simulink model "multi_model2015a"  (R2015a)
settings: Solver=ode3  SolverMode=SingleTasking  StartTime=0.0  StopTime=inf  FixedStep=0.01  RelTol=1e-3
values from neighbouring files (symbols this model uses):
  s = serial (serPort)    [UART_Connector.m]
undefined symbols (not defined in the file or in its folder): deg, rad
libraries: simulink x12, aerolibconvert2 x2, aerolibobsolete x1, aerolibatmos2 x1, aerolibnav x1, aerolibanimutils x1
settings Model: Creator=ADAM  LastModifiedBy=theth
settings DataIOCC: MaxDataPoints=1  SaveFormat=Structure  SignalLoggingSaveFormat=ModelDataLogs  SaveOutput=off  SignalLogging=off  DSMLogging=off  SaveTime=off  OutputSaveName=model_out  SignalLoggingName=model_out
settings OptimizationCC: ExpressionDepthLimit=2147483647
settings DebuggingCC: UnderspecifiedInitializationDetection=Classic  MergeDetectMultiDrivingBlocksExec=none  SolverPrmCheckMsg=warning  MultiTaskDSMMsg=warning  MultiTaskCondExecSysMsg=none  StateNameClashWarn=warning
settings HardwareCC: ProdBitPerLong=64  ProdBitPerPointer=64  ProdIntDivRoundTo=Zero  ProdEndianess=LittleEndian  ProdWordSize=64  ProdHWDeviceType=Intel->x86-64  TargetBitPerLong=64  TargetBitPerPointer=64  TargetIntDivRoundTo=Zero  TargetEndianess=LittleEndian  TargetWordSize=64  TargetHWDeviceType=Intel->x86-64
settings ModelReferenceCC: EnableParallelModelReferenceBuilds=on
settings RTWCC: SystemTargetFile=rtwin.tlc  TemplateMakefile=rtwin.tmf  Description=Simulink Desktop Real-Time  RTWCompilerOptimization=on
settings CodeAppCC: MaxIdLength=95
settings RTWinTargetCC: TargetPreCompLibLocation=D:\Matlab\toolbox\sldrt\lib\win64  GeneratePreprocessorConditionals=Use local settings  UseToolchainInfoCompliant=off  ExtModeMexFile=sldrtext

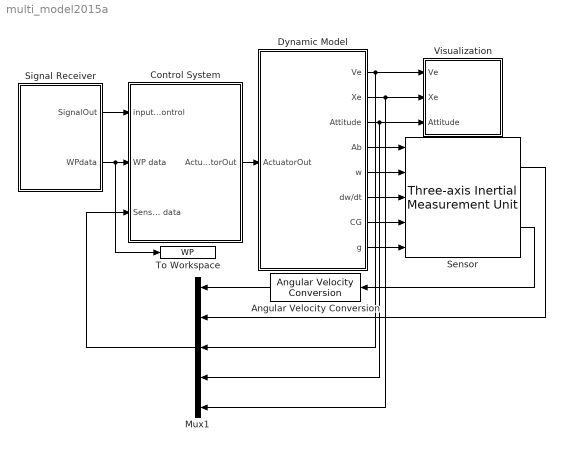
== system multi_model2015a ==
  Angular Velocity Conversion : aerolibconvert2/Angular Velocity Conversion  IU=rad/s  OU=deg/s
  Control System : Subsystem
      settings: CopyFcn=set_param(gcb,'BackgroundColor','green');
  Dynamic Model : Subsystem
      settings: CopyFcn=set_param(gcb,'BackgroundColor','orange');
  Mux1 : Mux  Inputs=5
  Sensor : aerolibnav/Three-axis Inertial Measurement Unit  units=Metric (MKS)  imu=[0 0 0]  dtype_a=off  w_a=190  z_a=0.707  a_sf_cc=[0.98 0 0; 0 0.98 0; 0 0 -0.98]  a_bias=[0 0 0]  a_sat="[-19.62  -19.62  -19.62 19.62 19.62 19.62]"  dtype_g=off  w_g=190  z_g=0.707  g_sf_cc=[.98 0 0; 0 .98 0; 0 0 .98]  g_bias=[0 0 0]  g_sens=[0 0 0]  g_sat="[-4.36  -4.36  -4.36 4.36 4.36 4.36]"  i_rand=on  i_seeds=[348631 366719 978432 189621 128794 214632]  i_pow=[0.000039 0.000039 0.000039 0.000000087 0.000000087 0.000000087]  i_Ts=0.01
  Signal Receiver : Subsystem
  To Workspace : ToWorkspace  VariableName=WP  SaveFormat=Structure  SampleTime=-1
  Visualization : Subsystem
  wires:
  Sensor/2 -> Angular Velocity Conversion/1
  Dynamic Model/2(Xe) -> Mux1/5, Visualization/2(Xe)
  Dynamic Model/3(Attitude) -> Mux1/4, Visualization/3(Attitude)
  Dynamic Model/4(Ab) -> Sensor/1
  Dynamic Model/5(w) -> Sensor/2
  Dynamic Model/6(dw/dt) -> Sensor/3
  Control System/1(ActuatorOut) -> Dynamic Model/1(ActuatorOut)
  Signal Receiver/1(SignalOut) -> Control System/1(inputControl)
  Dynamic Model/7(CG) -> Sensor/4
  Dynamic Model/8(g) -> Sensor/5
  Dynamic Model/1(Ve) -> Mux1/3, Visualization/1(Ve)
  Mux1/1 -> Control System/3(Sensors raw data)
  Angular Velocity Conversion/1 -> Mux1/1
  Sensor/1 -> Mux1/2
  Signal Receiver/2(WPdata) -> To Workspace/1, Control System/2(WP data)

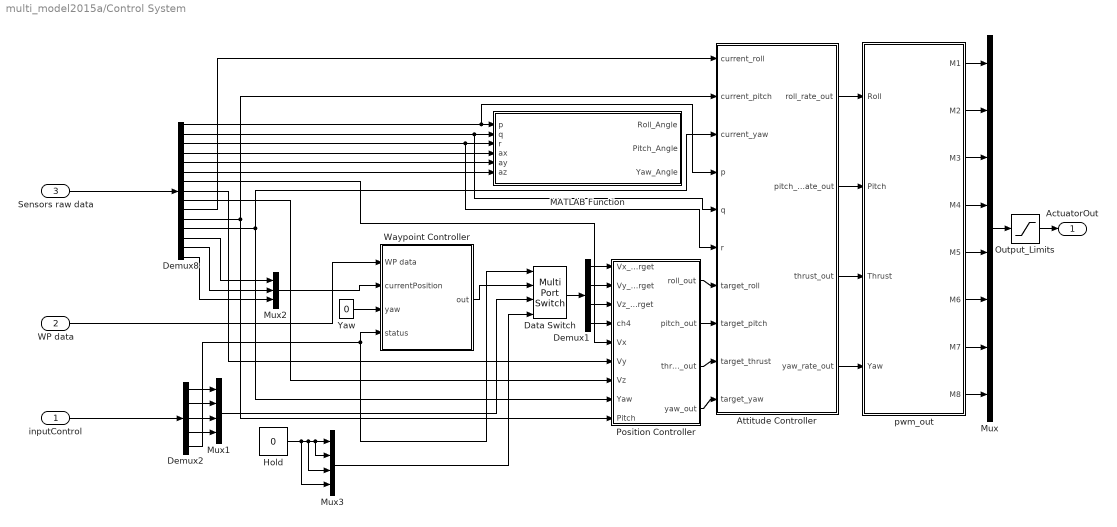
== system multi_model2015a/Control System ==
  inputControl : Inport
  WP data : Inport  Port=2
  Sensors raw data : Inport  Port=3
  Attitude Controller : Subsystem
  Data Switch : MultiPortSwitch  DataPortOrder=Zero-based contiguous
  Demux1 : Demux
  Demux2 : Demux  Outputs=5
  Demux8 : Demux  Outputs=15
  Hold : Constant  Value=0
  MATLAB Function : MATLAB Function  TreatAsAtomicUnit=on
      settings: PermitHierarchicalResolution=ParametersOnly
  Mux : Mux  Inputs=8
  Mux1 : Mux
  Mux2 : Mux  Inputs=3
  Mux3 : Mux
  Output_Limits : Saturate  UpperLimit=2000  LowerLimit=1000
  Position Controller : Subsystem
  Waypoint Controller : Subsystem
  Yaw : Constant  Value=0
  pwm_out : MATLAB Function  TreatAsAtomicUnit=on
      settings: PermitHierarchicalResolution=ParametersOnly
  ActuatorOut : Outport
  wires:
  pwm_out/8(M8) -> Mux/8
  pwm_out/7(M7) -> Mux/7
  pwm_out/6(M6) -> Mux/6
  pwm_out/5(M5) -> Mux/5
  pwm_out/4(M4) -> Mux/4
  pwm_out/3(M3) -> Mux/3
  pwm_out/2(M2) -> Mux/2
  pwm_out/1(M1) -> Mux/1
  Mux/1 -> Output_Limits/1
  Output_Limits/1 -> ActuatorOut/1
  Attitude Controller/3(thrust_out) -> pwm_out/3(Thrust)
  Attitude Controller/1(roll_rate_out) -> pwm_out/1(Roll)
  Attitude Controller/2(pitch_rate_out) -> pwm_out/2(Pitch)
  Attitude Controller/4(yaw_rate_out) -> pwm_out/4(Yaw)
  Position Controller/1(roll_out) -> Attitude Controller/7(target_roll)
  Position Controller/2(pitch_out) -> Attitude Controller/8(target_pitch)
  Position Controller/3(thrust_out) -> Attitude Controller/9(target_thrust)
  Position Controller/4(yaw_out) -> Attitude Controller/10(target_yaw)
  Demux1/3 -> Position Controller/3(Vz_target)
  Demux1/4 -> Position Controller/4(ch4)
  Demux1/1 -> Position Controller/1(Vx_target)
  Demux1/2 -> Position Controller/2(Vy_target)
  Demux8/1 -> Attitude Controller/4(p), MATLAB Function/1(p)
  Demux8/2 -> MATLAB Function/2(q), Attitude Controller/5(q)
  Demux8/3 -> MATLAB Function/3(r), Attitude Controller/6(r)
  Demux8/4 -> MATLAB Function/4(ax)
  Demux8/5 -> MATLAB Function/5(ay)
  Demux8/6 -> MATLAB Function/6(az)
  Demux8/7 -> Position Controller/5(Vx)
  Demux8/8 -> Position Controller/6(Vy)
  Demux8/9 -> Position Controller/7("Vz ")
  Demux8/12 -> Position Controller/8(Yaw), Attitude Controller/3(current_yaw)
  Demux8/11 -> Position Controller/9(Pitch), Attitude Controller/2(current_pitch)
  Demux8/10 -> Attitude Controller/1(current_roll)
  Yaw/1 -> Waypoint Controller/3(yaw)
  WP data/1 -> Waypoint Controller/1(WP data)
  Sensors raw data/1 -> Demux8/1
  Demux8/13 -> Mux2/1
  Demux8/14 -> Mux2/2
  Demux8/15 -> Mux2/3
  Mux2/1 -> Waypoint Controller/2(currentPosition)
  inputControl/1 -> Demux2/1
  Demux2/3 -> Mux1/3
  Demux2/2 -> Mux1/2
  Demux2/1 -> Mux1/1
  Demux2/4 -> Mux1/4
  Demux2/5 -> Data Switch/1, Waypoint Controller/4(status)
  Data Switch/1 -> Demux1/1
  Hold/1 -> Mux3/4, Mux3/3, Mux3/2, Mux3/1
  Mux3/1 -> Data Switch/4
  Waypoint Controller/1(out) -> Data Switch/2
  Mux1/1 -> Data Switch/3

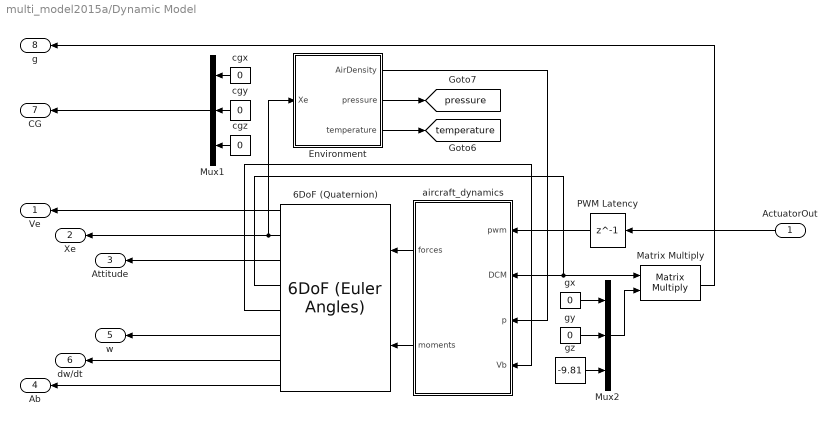
== system multi_model2015a/Dynamic Model ==
  ActuatorOut : Inport
  6DoF (Quaternion) : aerolibobsolete/6DoF (Euler Angles)  units=Metric (MKS)  mtype=Fixed  rep=Quaternion  xme_0=[0 0 0]  Vm_0=[0 0 0]  eul_0=[0 0 0]  pm_0=[0 0 0]  mass_0=1  mass_e=0  mass_f=0  inertia=[0.016, 0, 0; 0, 0.016, 0; 0, 0, 0.031]  inertia_e=eye(3)  inertia_f=eye(3)  k_quat=1.0
  Environment : Subsystem  TreatAsAtomicUnit=on
  Matrix Multiply : Product  Multiplication=Matrix(*)
  Mux1 : Mux  Inputs=3
  Mux2 : Mux  Inputs=3
  PWM Latency : Delay  DelayLength=1
  aircraft_dynamics : MATLAB Function  TreatAsAtomicUnit=on
      settings: PermitHierarchicalResolution=ParametersOnly
  cgx : Constant  Value=0
  cgy : Constant  Value=0
  cgz : Constant  Value=0
  gx : Constant  Value=0
  gy : Constant  Value=0
  gz : Constant  Value=-9.81
  Ve : Outport
  Xe : Outport  Port=2
  Attitude : Outport  Port=3
  Ab : Outport  Port=4
  w : Outport  Port=5
  dw/dt : Outport  Port=6
  CG : Outport  Port=7
  g : Outport  Port=8
  tag scope: pressure=global, temperature=global
  wires:
  6DoF (Quaternion)/4 -> Matrix Multiply/1, aircraft_dynamics/2(DCM)
  PWM Latency/1 -> aircraft_dynamics/1(pwm)
  6DoF (Quaternion)/2 -> Xe/1, Environment/1(Xe)
  6DoF (Quaternion)/5 -> aircraft_dynamics/4(Vb)
  aircraft_dynamics/2(moments) -> 6DoF (Quaternion)/2
  aircraft_dynamics/1(forces) -> 6DoF (Quaternion)/1
  6DoF (Quaternion)/6 -> w/1
  6DoF (Quaternion)/1 -> Ve/1
  6DoF (Quaternion)/3 -> Attitude/1
  Environment/1(AirDensity) -> aircraft_dynamics/3(p)
  Environment/3(temperature) -> [temperature]
  Environment/2(pressure) -> [pressure]
  ActuatorOut/1 -> PWM Latency/1
  6DoF (Quaternion)/8 -> Ab/1
  6DoF (Quaternion)/7 -> dw/dt/1
  cgy/1 -> Mux1/2
  gy/1 -> Mux2/2
  gx/1 -> Mux2/1
  cgx/1 -> Mux1/1
  cgz/1 -> Mux1/3
  gz/1 -> Mux2/3
  Mux2/1 -> Matrix Multiply/2
  Mux1/1 -> CG/1
  Matrix Multiply/1 -> g/1

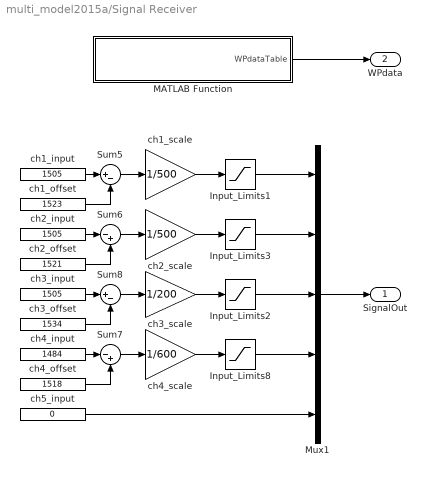
== system multi_model2015a/Signal Receiver ==
  Input_Limits1 : Saturate  UpperLimit=1  LowerLimit=-1
  Input_Limits2 : Saturate  UpperLimit=2.5  LowerLimit=-2.5
  Input_Limits3 : Saturate  UpperLimit=1  LowerLimit=-1
  Input_Limits8 : Saturate  UpperLimit=1  LowerLimit=-1
  MATLAB Function : MATLAB Function  TreatAsAtomicUnit=on
      settings: PermitHierarchicalResolution=ParametersOnly
  Mux1 : Mux  Inputs=5
  Sum5 : Sum  Inputs=|+-
  Sum6 : Sum  Inputs=|-+
  Sum7 : Sum  Inputs=|-+
  Sum8 : Sum  Inputs=|+-
  ch1_input : Constant  Value=1505
  ch1_offset : Constant  Value=1523
  ch1_scale : Gain  Gain=1/500
  ch2_input : Constant  Value=1505
  ch2_offset : Constant  Value=1521
  ch2_scale : Gain  Gain=1/500
  ch3_input : Constant  Value=1505
  ch3_offset : Constant  Value=1534
  ch3_scale : Gain  Gain=1/200
  ch4_input : Constant  Value=1484
  ch4_offset : Constant  Value=1518
  ch4_scale : Gain  Gain=1/600
  ch5_input : Constant  Value=0
  SignalOut : Outport
  WPdata : Outport  Port=2
  wires:
  Input_Limits8/1 -> Mux1/4
  Input_Limits2/1 -> Mux1/3
  Input_Limits1/1 -> Mux1/1
  Input_Limits3/1 -> Mux1/2
  Mux1/1 -> SignalOut/1
  MATLAB Function/1(WPdataTable) -> WPdata/1
  Sum6/1 -> ch2_scale/1
  Sum7/1 -> ch4_scale/1
  ch3_input/1 -> Sum8/1
  ch4_input/1 -> Sum7/1
  ch2_input/1 -> Sum6/1
  ch1_input/1 -> Sum5/1
  Sum5/1 -> ch1_scale/1
  Sum8/1 -> ch3_scale/1
  ch1_offset/1 -> Sum5/2
  ch2_offset/1 -> Sum6/2
  ch4_offset/1 -> Sum7/2
  ch4_scale/1 -> Input_Limits8/1
  ch3_offset/1 -> Sum8/2
  ch3_scale/1 -> Input_Limits2/1
  ch1_scale/1 -> Input_Limits1/1
  ch2_scale/1 -> Input_Limits3/1
  ch5_input/1 -> Mux1/5

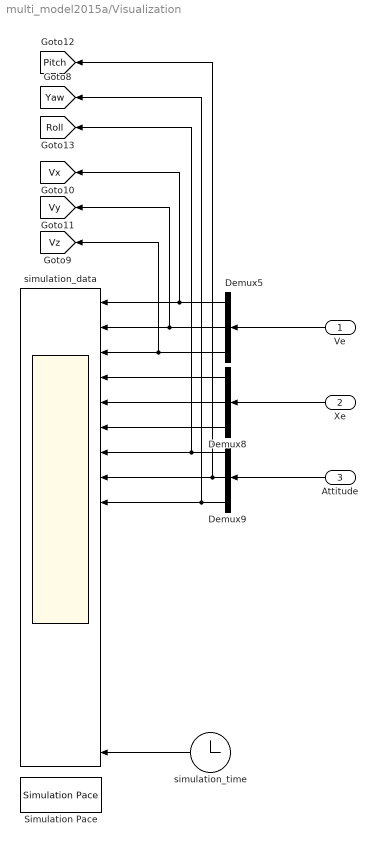
== system multi_model2015a/Visualization ==
  Ve : Inport
  Xe : Inport  Port=2
  Attitude : Inport  Port=3
  Demux5 : Demux  Outputs=3
  Demux8 : Demux  Outputs=3
  Demux9 : Demux  Outputs=3
  Simulation Pace : aerolibanimutils/Simulation Pace  SimulationPace=1  SleepMode=MATLAB Thread  OutputPaceError=off  SampleTime=-1
      settings: AttributesFormatString=%<SimulationPace> sec/sec
  simulation_data : Scope  NumInputPorts=19
      settings: TimeRange=auto  MaxDataPoints=5000  SaveToWorkspace=off  SaveName=ScopeData7  YMin=0.261~-0.28~15.25~34~-22~1725~-0.02~-0.04~0.01~-0.15~-0.1~-0.03~-0.4~-0.4~-10~-1~-5~-5~-5  YMax=0.275~-0.24~15.5~39~-17~1975~0.04~0.04~0.09~0.15~0.125~0.03~0.4~0.4~-9.2~1~5~5~5  SampleTime=-1
  simulation_time : Clock
  tag scope: Pitch=global, Roll=global, Vx=global, Vy=global, Vz=global, Yaw=global
  wires:
  Xe/1 -> Demux8/1
  Demux9/1 -> simulation_data/7, [Roll]
  Demux9/2 -> simulation_data/8, [Pitch]
  Attitude/1 -> Demux9/1
  Demux8/1 -> simulation_data/4
  Demux8/2 -> simulation_data/5
  Demux8/3 -> simulation_data/6
  Demux9/3 -> simulation_data/9, [Yaw]
  simulation_time/1 -> simulation_data/19
  Ve/1 -> Demux5/1
  Demux5/1 -> simulation_data/1, [Vx]
  Demux5/2 -> simulation_data/2, [Vy]
  Demux5/3 -> [Vz], simulation_data/3

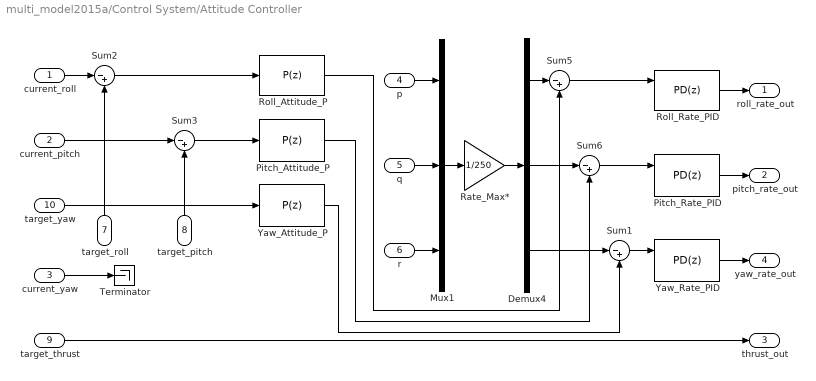
== system multi_model2015a/Control System/Attitude Controller ==
  current_roll : Inport
  current_pitch : Inport  Port=2
  current_yaw : Inport  Port=3
  p : Inport  Port=4
  q : Inport  Port=5
  r : Inport  Port=6
  target_roll : Inport  Port=7
  target_pitch : Inport  Port=8
  target_thrust : Inport  Port=9
  target_yaw : Inport  Port=10
  Demux4 : Demux  Outputs=3
  Mux1 : Mux  Inputs=3
  Pitch_Attitude_P : simulink/Continuous/PID Controller  Controller=P  TimeDomain=Discrete-time  SampleTime=-1  IntegratorMethod=Forward Euler  FilterMethod=Forward Euler  Form=Parallel  UseFilter=on  ControllerParametersSource=internal  P=1  I=0  D=0  N=100  InitialConditionSource=internal  InitialConditionForIntegrator=0  InitialConditionForFilter=0  ExternalReset=either  LimitOutput=on  UpperSaturationLimit=1  LowerSaturationLimit=-1  LinearizeAsGain=on  AntiWindupMode=none  Kb=1  TrackingMode=off  Kt=1  PParamMin=[]  PParamMax=[]  IParamMin=[]  IParamMax=[]  DParamMin=[]  DParamMax=[]  NParamMin=[]  NParamMax=[]  KbParamMin=[]  KbParamMax=[]  KtParamMin=[]  KtParamMax=[]  POutMin=[]  POutMax=[]  IOutMin=[]  IOutMax=[]  DOutMin=[]  DOutMax=[]  NOutMin=[]  NOutMax=[]  KbOutMin=[]  KbOutMax=[]  KtOutMin=[]  KtOutMax=[]  IntegratorOutMin=[]  IntegratorOutMax=[]  FilterOutMin=[]  FilterOutMax=[]  SumOutMin=[]  SumOutMax=[]  SumI1OutMin=[]  SumI1OutMax=[]  SumI2OutMin=[]  SumI2OutMax=[]  SumI3OutMin=[]  SumI3OutMax=[]  SumDOutMin=[]  SumDOutMax=[]  SaturationOutMin=[]  SaturationOutMax=[]  IntegratorContinuousStateAttributes=''  IntegratorStateMustResolveToSignalObject=off  IntegratorRTWStateStorageClass=Auto  FilterContinuousStateAttributes=''  FilterStateMustResolveToSignalObject=off  FilterRTWStateStorageClass=Auto  DifferentiatorICPrevScaledInput=0  DifferentiatorOutMin=[]  DifferentiatorOutMax=[]
  Pitch_Rate_PID : simulink/Continuous/PID Controller  Controller=PD  TimeDomain=Discrete-time  SampleTime=-1  IntegratorMethod=Forward Euler  FilterMethod=Forward Euler  Form=Parallel  UseFilter=off  ControllerParametersSource=internal  P=2  I=0  D=0.01  N=20  InitialConditionSource=internal  InitialConditionForIntegrator=0  InitialConditionForFilter=0  ExternalReset=either  LimitOutput=on  UpperSaturationLimit=1  LowerSaturationLimit=-1  LinearizeAsGain=on  AntiWindupMode=none  Kb=1  TrackingMode=off  Kt=1  PParamMin=[]  PParamMax=[]  IParamMin=[]  IParamMax=[]  DParamMin=[]  DParamMax=[]  NParamMin=[]  NParamMax=[]  KbParamMin=[]  KbParamMax=[]  KtParamMin=[]  KtParamMax=[]  POutMin=[]  POutMax=[]  IOutMin=[]  IOutMax=[]  DOutMin=[]  DOutMax=[]  NOutMin=[]  NOutMax=[]  KbOutMin=[]  KbOutMax=[]  KtOutMin=[]  KtOutMax=[]  IntegratorOutMin=[]  IntegratorOutMax=[]  FilterOutMin=[]  FilterOutMax=[]  SumOutMin=[]  SumOutMax=[]  SumI1OutMin=[]  SumI1OutMax=[]  SumI2OutMin=[]  SumI2OutMax=[]  SumI3OutMin=[]  SumI3OutMax=[]  SumDOutMin=[]  SumDOutMax=[]  SaturationOutMin=[]  SaturationOutMax=[]  IntegratorContinuousStateAttributes=''  IntegratorStateMustResolveToSignalObject=off  IntegratorRTWStateStorageClass=Auto  FilterContinuousStateAttributes=''  FilterStateMustResolveToSignalObject=off  FilterRTWStateStorageClass=Auto  DifferentiatorICPrevScaledInput=0  DifferentiatorOutMin=[]  DifferentiatorOutMax=[]
  Rate_Max* : Gain  Gain=1/250
  Roll_Attitude_P : simulink/Continuous/PID Controller  Controller=P  TimeDomain=Discrete-time  SampleTime=-1  IntegratorMethod=Forward Euler  FilterMethod=Forward Euler  Form=Parallel  UseFilter=on  ControllerParametersSource=internal  P=1  I=0  D=0  N=100  InitialConditionSource=internal  InitialConditionForIntegrator=0  InitialConditionForFilter=0  ExternalReset=either  LimitOutput=on  UpperSaturationLimit=1  LowerSaturationLimit=-1  LinearizeAsGain=on  AntiWindupMode=none  Kb=1  TrackingMode=off  Kt=1  PParamMin=[]  PParamMax=[]  IParamMin=[]  IParamMax=[]  DParamMin=[]  DParamMax=[]  NParamMin=[]  NParamMax=[]  KbParamMin=[]  KbParamMax=[]  KtParamMin=[]  KtParamMax=[]  POutMin=[]  POutMax=[]  IOutMin=[]  IOutMax=[]  DOutMin=[]  DOutMax=[]  NOutMin=[]  NOutMax=[]  KbOutMin=[]  KbOutMax=[]  KtOutMin=[]  KtOutMax=[]  IntegratorOutMin=[]  IntegratorOutMax=[]  FilterOutMin=[]  FilterOutMax=[]  SumOutMin=[]  SumOutMax=[]  SumI1OutMin=[]  SumI1OutMax=[]  SumI2OutMin=[]  SumI2OutMax=[]  SumI3OutMin=[]  SumI3OutMax=[]  SumDOutMin=[]  SumDOutMax=[]  SaturationOutMin=[]  SaturationOutMax=[]  IntegratorContinuousStateAttributes=''  IntegratorStateMustResolveToSignalObject=off  IntegratorRTWStateStorageClass=Auto  FilterContinuousStateAttributes=''  FilterStateMustResolveToSignalObject=off  FilterRTWStateStorageClass=Auto  DifferentiatorICPrevScaledInput=0  DifferentiatorOutMin=[]  DifferentiatorOutMax=[]
  Roll_Rate_PID : simulink/Continuous/PID Controller  Controller=PD  TimeDomain=Discrete-time  SampleTime=-1  IntegratorMethod=Forward Euler  FilterMethod=Forward Euler  Form=Parallel  UseFilter=off  ControllerParametersSource=internal  P=2  I=0  D=0.01  N=20  InitialConditionSource=internal  InitialConditionForIntegrator=0  InitialConditionForFilter=0  ExternalReset=either  LimitOutput=on  UpperSaturationLimit=1  LowerSaturationLimit=-1  LinearizeAsGain=on  AntiWindupMode=none  Kb=1  TrackingMode=off  Kt=1  PParamMin=[]  PParamMax=[]  IParamMin=[]  IParamMax=[]  DParamMin=[]  DParamMax=[]  NParamMin=[]  NParamMax=[]  KbParamMin=[]  KbParamMax=[]  KtParamMin=[]  KtParamMax=[]  POutMin=[]  POutMax=[]  IOutMin=[]  IOutMax=[]  DOutMin=[]  DOutMax=[]  NOutMin=[]  NOutMax=[]  KbOutMin=[]  KbOutMax=[]  KtOutMin=[]  KtOutMax=[]  IntegratorOutMin=[]  IntegratorOutMax=[]  FilterOutMin=[]  FilterOutMax=[]  SumOutMin=[]  SumOutMax=[]  SumI1OutMin=[]  SumI1OutMax=[]  SumI2OutMin=[]  SumI2OutMax=[]  SumI3OutMin=[]  SumI3OutMax=[]  SumDOutMin=[]  SumDOutMax=[]  SaturationOutMin=[]  SaturationOutMax=[]  IntegratorContinuousStateAttributes=''  IntegratorStateMustResolveToSignalObject=off  IntegratorRTWStateStorageClass=Auto  FilterContinuousStateAttributes=''  FilterStateMustResolveToSignalObject=off  FilterRTWStateStorageClass=Auto  DifferentiatorICPrevScaledInput=0  DifferentiatorOutMin=[]  DifferentiatorOutMax=[]
  Sum{1..3,5..6} (5 alike) : Sum  Inputs=|-+
  Terminator : Terminator
  Yaw_Attitude_P : simulink/Continuous/PID Controller  Controller=P  TimeDomain=Discrete-time  SampleTime=-1  IntegratorMethod=Forward Euler  FilterMethod=Forward Euler  Form=Parallel  UseFilter=on  ControllerParametersSource=internal  P=1  I=0  D=0  N=100  InitialConditionSource=internal  InitialConditionForIntegrator=0  InitialConditionForFilter=0  ExternalReset=either  LimitOutput=on  UpperSaturationLimit=1  LowerSaturationLimit=-1  LinearizeAsGain=on  AntiWindupMode=none  Kb=1  TrackingMode=off  Kt=1  PParamMin=[]  PParamMax=[]  IParamMin=[]  IParamMax=[]  DParamMin=[]  DParamMax=[]  NParamMin=[]  NParamMax=[]  KbParamMin=[]  KbParamMax=[]  KtParamMin=[]  KtParamMax=[]  POutMin=[]  POutMax=[]  IOutMin=[]  IOutMax=[]  DOutMin=[]  DOutMax=[]  NOutMin=[]  NOutMax=[]  KbOutMin=[]  KbOutMax=[]  KtOutMin=[]  KtOutMax=[]  IntegratorOutMin=[]  IntegratorOutMax=[]  FilterOutMin=[]  FilterOutMax=[]  SumOutMin=[]  SumOutMax=[]  SumI1OutMin=[]  SumI1OutMax=[]  SumI2OutMin=[]  SumI2OutMax=[]  SumI3OutMin=[]  SumI3OutMax=[]  SumDOutMin=[]  SumDOutMax=[]  SaturationOutMin=[]  SaturationOutMax=[]  IntegratorContinuousStateAttributes=''  IntegratorStateMustResolveToSignalObject=off  IntegratorRTWStateStorageClass=Auto  FilterContinuousStateAttributes=''  FilterStateMustResolveToSignalObject=off  FilterRTWStateStorageClass=Auto  DifferentiatorICPrevScaledInput=0  DifferentiatorOutMin=[]  DifferentiatorOutMax=[]
  Yaw_Rate_PID : simulink/Continuous/PID Controller  Controller=PD  TimeDomain=Discrete-time  SampleTime=-1  IntegratorMethod=Forward Euler  FilterMethod=Forward Euler  Form=Parallel  UseFilter=off  ControllerParametersSource=internal  P=4.5  I=0  D=0.1  N=20  InitialConditionSource=internal  InitialConditionForIntegrator=0  InitialConditionForFilter=0  ExternalReset=either  LimitOutput=on  UpperSaturationLimit=1  LowerSaturationLimit=-1  LinearizeAsGain=on  AntiWindupMode=none  Kb=1  TrackingMode=off  Kt=1  PParamMin=[]  PParamMax=[]  IParamMin=[]  IParamMax=[]  DParamMin=[]  DParamMax=[]  NParamMin=[]  NParamMax=[]  KbParamMin=[]  KbParamMax=[]  KtParamMin=[]  KtParamMax=[]  POutMin=[]  POutMax=[]  IOutMin=[]  IOutMax=[]  DOutMin=[]  DOutMax=[]  NOutMin=[]  NOutMax=[]  KbOutMin=[]  KbOutMax=[]  KtOutMin=[]  KtOutMax=[]  IntegratorOutMin=[]  IntegratorOutMax=[]  FilterOutMin=[]  FilterOutMax=[]  SumOutMin=[]  SumOutMax=[]  SumI1OutMin=[]  SumI1OutMax=[]  SumI2OutMin=[]  SumI2OutMax=[]  SumI3OutMin=[]  SumI3OutMax=[]  SumDOutMin=[]  SumDOutMax=[]  SaturationOutMin=[]  SaturationOutMax=[]  IntegratorContinuousStateAttributes=''  IntegratorStateMustResolveToSignalObject=off  IntegratorRTWStateStorageClass=Auto  FilterContinuousStateAttributes=''  FilterStateMustResolveToSignalObject=off  FilterRTWStateStorageClass=Auto  DifferentiatorICPrevScaledInput=0  DifferentiatorOutMin=[]  DifferentiatorOutMax=[]
  roll_rate_out : Outport
  pitch_rate_out : Outport  Port=2
  thrust_out : Outport  Port=3
  yaw_rate_out : Outport  Port=4
  wires:
  Sum5/1 -> Roll_Rate_PID/1
  Rate_Max*/1 -> Demux4/1
  Demux4/2 -> Sum6/1
  Demux4/1 -> Sum5/1
  Sum1/1 -> Yaw_Rate_PID/1
  Sum6/1 -> Pitch_Rate_PID/1
  Demux4/3 -> Sum1/1
  Mux1/1 -> Rate_Max*/1
  Sum2/1 -> Roll_Attitude_P/1
  Sum3/1 -> Pitch_Attitude_P/1
  current_pitch/1 -> Sum3/1
  current_roll/1 -> Sum2/1
  p/1 -> Mux1/1
  q/1 -> Mux1/2
  r/1 -> Mux1/3
  Yaw_Attitude_P/1 -> Sum1/2
  Pitch_Attitude_P/1 -> Sum6/2
  Roll_Attitude_P/1 -> Sum5/2
  target_roll/1 -> Sum2/2
  target_pitch/1 -> Sum3/2
  target_thrust/1 -> thrust_out/1
  Yaw_Rate_PID/1 -> yaw_rate_out/1
  Pitch_Rate_PID/1 -> pitch_rate_out/1
  Roll_Rate_PID/1 -> roll_rate_out/1
  target_yaw/1 -> Yaw_Attitude_P/1
  current_yaw/1 -> Terminator/1

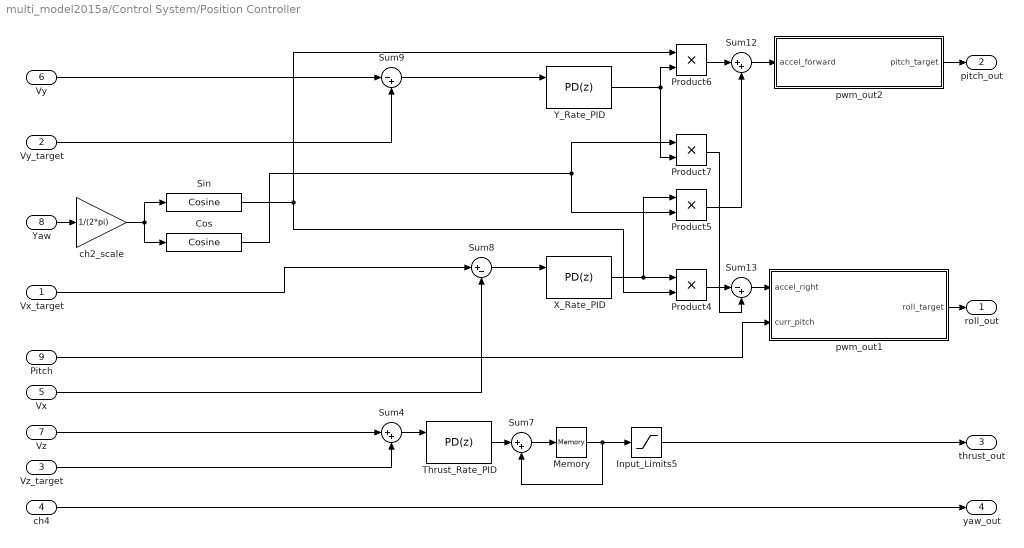
== system multi_model2015a/Control System/Position Controller ==
  Vx_target : Inport
  Vy_target : Inport  Port=2
  Vz_target : Inport  Port=3
  ch4 : Inport  Port=4
  Vx : Inport  Port=5
  Vy : Inport  Port=6
  "Vz " : Inport  Port=7
  Yaw : Inport  Port=8
  Pitch : Inport  Port=9
  Cos : simulink/Lookup Tables/Cosine  Formula=cos(2*pi*u)  NumDataPoints=(2^5)+1  OutputWordLength=16  InternalRulePriority=Speed
  Input_Limits5 : Saturate  UpperLimit=1  LowerLimit=0
  Memory : Memory  InheritSampleTime=on  LinearizeMemory=on
  Product{4..7} (4 alike) : Product
  Sin : simulink/Lookup Tables/Cosine  Formula=sin(2*pi*u)  NumDataPoints=(2^5)+1  OutputWordLength=16  InternalRulePriority=Speed
  Sum12 : Sum  Inputs=|++
  Sum13 : Sum  Inputs=|-+
  Sum4 : Sum  Inputs=|++
  Sum7 : Sum  Inputs=|++
  Sum8 : Sum  Inputs=|+-
  Sum9 : Sum  Inputs=|-+
  Thrust_Rate_PID : simulink/Continuous/PID Controller  Controller=PD  TimeDomain=Discrete-time  SampleTime=-1  IntegratorMethod=Forward Euler  FilterMethod=Forward Euler  Form=Parallel  UseFilter=off  ControllerParametersSource=internal  P=0.1  I=0.1  D=0.01  N=20  InitialConditionSource=internal  InitialConditionForIntegrator=0  InitialConditionForFilter=0  ExternalReset=either  LimitOutput=on  UpperSaturationLimit=1  LowerSaturationLimit=-1  LinearizeAsGain=on  AntiWindupMode=none  Kb=1  TrackingMode=off  Kt=1  PParamMin=[]  PParamMax=[]  IParamMin=[]  IParamMax=[]  DParamMin=[]  DParamMax=[]  NParamMin=[]  NParamMax=[]  KbParamMin=[]  KbParamMax=[]  KtParamMin=[]  KtParamMax=[]  POutMin=[]  POutMax=[]  IOutMin=[]  IOutMax=[]  DOutMin=[]  DOutMax=[]  NOutMin=[]  NOutMax=[]  KbOutMin=[]  KbOutMax=[]  KtOutMin=[]  KtOutMax=[]  IntegratorOutMin=[]  IntegratorOutMax=[]  FilterOutMin=[]  FilterOutMax=[]  SumOutMin=[]  SumOutMax=[]  SumI1OutMin=[]  SumI1OutMax=[]  SumI2OutMin=[]  SumI2OutMax=[]  SumI3OutMin=[]  SumI3OutMax=[]  SumDOutMin=[]  SumDOutMax=[]  SaturationOutMin=[]  SaturationOutMax=[]  IntegratorContinuousStateAttributes=''  IntegratorStateMustResolveToSignalObject=off  IntegratorRTWStateStorageClass=Auto  FilterContinuousStateAttributes=''  FilterStateMustResolveToSignalObject=off  FilterRTWStateStorageClass=Auto  DifferentiatorICPrevScaledInput=0  DifferentiatorOutMin=[]  DifferentiatorOutMax=[]
  X_Rate_PID : simulink/Continuous/PID Controller  Controller=PD  TimeDomain=Discrete-time  SampleTime=-1  IntegratorMethod=Forward Euler  FilterMethod=Forward Euler  Form=Parallel  UseFilter=off  ControllerParametersSource=internal  P=1  I=0.01  D=0.01  N=20  InitialConditionSource=internal  InitialConditionForIntegrator=0  InitialConditionForFilter=0  ExternalReset=either  LimitOutput=on  UpperSaturationLimit=1  LowerSaturationLimit=-1  LinearizeAsGain=on  AntiWindupMode=none  Kb=1  TrackingMode=off  Kt=1  PParamMin=[]  PParamMax=[]  IParamMin=[]  IParamMax=[]  DParamMin=[]  DParamMax=[]  NParamMin=[]  NParamMax=[]  KbParamMin=[]  KbParamMax=[]  KtParamMin=[]  KtParamMax=[]  POutMin=[]  POutMax=[]  IOutMin=[]  IOutMax=[]  DOutMin=[]  DOutMax=[]  NOutMin=[]  NOutMax=[]  KbOutMin=[]  KbOutMax=[]  KtOutMin=[]  KtOutMax=[]  IntegratorOutMin=[]  IntegratorOutMax=[]  FilterOutMin=[]  FilterOutMax=[]  SumOutMin=[]  SumOutMax=[]  SumI1OutMin=[]  SumI1OutMax=[]  SumI2OutMin=[]  SumI2OutMax=[]  SumI3OutMin=[]  SumI3OutMax=[]  SumDOutMin=[]  SumDOutMax=[]  SaturationOutMin=[]  SaturationOutMax=[]  IntegratorContinuousStateAttributes=''  IntegratorStateMustResolveToSignalObject=off  IntegratorRTWStateStorageClass=Auto  FilterContinuousStateAttributes=''  FilterStateMustResolveToSignalObject=off  FilterRTWStateStorageClass=Auto  DifferentiatorICPrevScaledInput=0  DifferentiatorOutMin=[]  DifferentiatorOutMax=[]
  Y_Rate_PID : simulink/Continuous/PID Controller  Controller=PD  TimeDomain=Discrete-time  SampleTime=-1  IntegratorMethod=Forward Euler  FilterMethod=Forward Euler  Form=Parallel  UseFilter=off  ControllerParametersSource=internal  P=1  I=0.01  D=0.01  N=20  InitialConditionSource=internal  InitialConditionForIntegrator=0  InitialConditionForFilter=0  ExternalReset=either  LimitOutput=on  UpperSaturationLimit=1  LowerSaturationLimit=-1  LinearizeAsGain=on  AntiWindupMode=none  Kb=1  TrackingMode=off  Kt=1  PParamMin=[]  PParamMax=[]  IParamMin=[]  IParamMax=[]  DParamMin=[]  DParamMax=[]  NParamMin=[]  NParamMax=[]  KbParamMin=[]  KbParamMax=[]  KtParamMin=[]  KtParamMax=[]  POutMin=[]  POutMax=[]  IOutMin=[]  IOutMax=[]  DOutMin=[]  DOutMax=[]  NOutMin=[]  NOutMax=[]  KbOutMin=[]  KbOutMax=[]  KtOutMin=[]  KtOutMax=[]  IntegratorOutMin=[]  IntegratorOutMax=[]  FilterOutMin=[]  FilterOutMax=[]  SumOutMin=[]  SumOutMax=[]  SumI1OutMin=[]  SumI1OutMax=[]  SumI2OutMin=[]  SumI2OutMax=[]  SumI3OutMin=[]  SumI3OutMax=[]  SumDOutMin=[]  SumDOutMax=[]  SaturationOutMin=[]  SaturationOutMax=[]  IntegratorContinuousStateAttributes=''  IntegratorStateMustResolveToSignalObject=off  IntegratorRTWStateStorageClass=Auto  FilterContinuousStateAttributes=''  FilterStateMustResolveToSignalObject=off  FilterRTWStateStorageClass=Auto  DifferentiatorICPrevScaledInput=0  DifferentiatorOutMin=[]  DifferentiatorOutMax=[]
  ch2_scale : Gain  Gain=1/(2*pi)
  pwm_out1 : MATLAB Function  TreatAsAtomicUnit=on
      settings: PermitHierarchicalResolution=ParametersOnly
  pwm_out2 : MATLAB Function  TreatAsAtomicUnit=on
      settings: PermitHierarchicalResolution=ParametersOnly
  roll_out : Outport
  pitch_out : Outport  Port=2
  thrust_out : Outport  Port=3
  yaw_out : Outport  Port=4
  wires:
  X_Rate_PID/1 -> Product4/1, Product5/1
  Y_Rate_PID/1 -> Product7/2, Product6/2
  Sum8/1 -> X_Rate_PID/1
  Vx_target/1 -> Sum8/1
  Sum12/1 -> pwm_out2/1(accel_forward)
  Cos/1 -> Product7/1, Product5/2
  Sin/1 -> Product6/1, Product4/2
  Yaw/1 -> ch2_scale/1
  Vy/1 -> Sum9/1
  Sum9/1 -> Y_Rate_PID/1
  Vx/1 -> Sum8/2
  pwm_out2/1(pitch_target) -> pitch_out/1
  pwm_out1/1(roll_target) -> roll_out/1
  ch4/1 -> yaw_out/1
  Product5/1 -> Sum12/2
  Product6/1 -> Sum12/1
  Sum13/1 -> pwm_out1/1(accel_right)
  Pitch/1 -> pwm_out1/2(curr_pitch)
  Product7/1 -> Sum13/2
  Product4/1 -> Sum13/1
  ch2_scale/1 -> Cos/1, Sin/1
  Sum4/1 -> Thrust_Rate_PID/1
  Memory/1 -> Input_Limits5/1, Sum7/2
  Sum7/1 -> Memory/1
  Thrust_Rate_PID/1 -> Sum7/1
  "Vz "/1 -> Sum4/1
  Vz_target/1 -> Sum4/2
  Input_Limits5/1 -> thrust_out/1
  Vy_target/1 -> Sum9/2

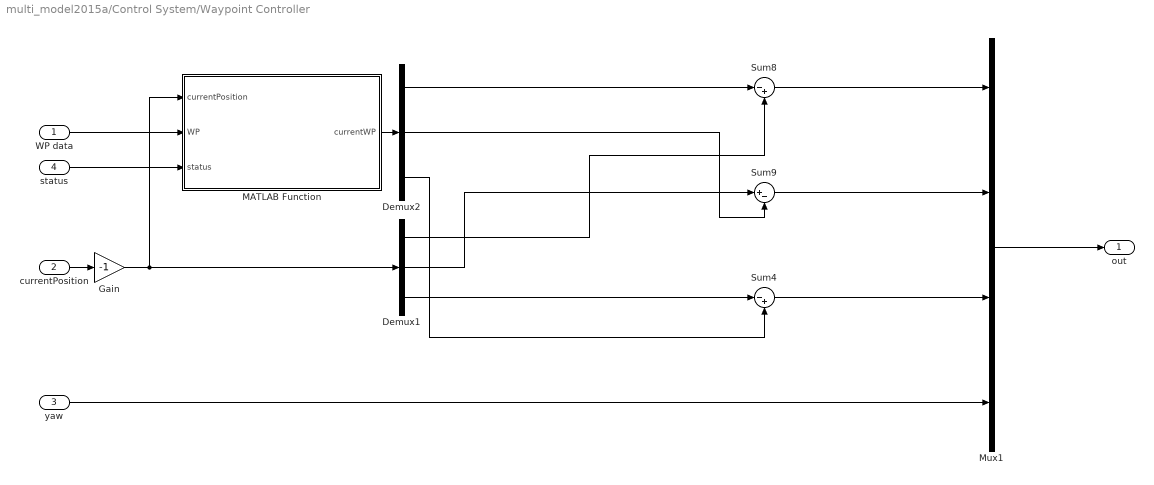
== system multi_model2015a/Control System/Waypoint Controller ==
  WP data : Inport
  currentPosition : Inport  Port=2
  yaw : Inport  Port=3
  status : Inport  Port=4
  Demux1 : Demux  Outputs=3
  Demux2 : Demux  Outputs=3
  Gain : Gain  Gain=-1
  MATLAB Function : MATLAB Function  TreatAsAtomicUnit=on
      settings: PermitHierarchicalResolution=ParametersOnly
  Mux1 : Mux
  Sum4 : Sum  Inputs=|-+
  Sum8 : Sum  Inputs=|-+
  Sum9 : Sum  Inputs=|+-
  out : Outport
  wires:
  Demux2/1 -> Sum8/1
  Demux1/2 -> Sum9/1
  Demux1/1 -> Sum8/2
  yaw/1 -> Mux1/4
  Demux1/3 -> Sum4/1
  Demux2/3 -> Sum4/2
  Mux1/1 -> out/1
  MATLAB Function/1(currentWP) -> Demux2/1
  Demux2/2 -> Sum9/2
  WP data/1 -> MATLAB Function/2(WP)
  status/1 -> MATLAB Function/3(status)
  Sum9/1 -> Mux1/2
  Sum4/1 -> Mux1/3
  Sum8/1 -> Mux1/1
  currentPosition/1 -> Gain/1
  Gain/1 -> MATLAB Function/1(currentPosition), Demux1/1

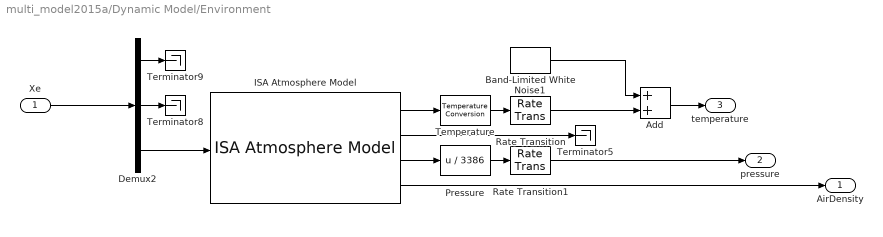
== system multi_model2015a/Dynamic Model/Environment ==
  Xe : Inport
  Add : Sum
  Band-Limited White Noise1 : simulink/Sources/Band-Limited White Noise  Cov=[0.0001]  Ts=0.5  seed=[23341]
  Demux2 : Demux  Outputs=3
  ISA Atmosphere Model : aerolibatmos2/ISA Atmosphere Model  custom=on  g=9.80665  gamma=1.4  R=287.0531  L=0.0065  h_trop=11000  h_strat=20000  rho0=1.225  P0=101325  T0=288.15  h0=0
  Pressure : Fcn  Expr=u / 3386
  Rate Transition : RateTransition  OutPortSampleTime=0.01
  Rate Transition1 : RateTransition  OutPortSampleTime=0.05
  Temperature : aerolibconvert2/Temperature Conversion  IU=K  OU=C
  Terminator5 : Terminator
  Terminator8 : Terminator
  Terminator9 : Terminator
  AirDensity : Outport
  pressure : Outport  Port=2
  temperature : Outport  Port=3
  wires:
  Demux2/2 -> Terminator8/1
  Demux2/1 -> Terminator9/1
  Demux2/3 -> ISA Atmosphere Model/1
  Xe/1 -> Demux2/1
  ISA Atmosphere Model/3 -> Pressure/1
  ISA Atmosphere Model/2 -> Terminator5/1
  ISA Atmosphere Model/4 -> AirDensity/1
  ISA Atmosphere Model/1 -> Temperature/1
  Temperature/1 -> Rate Transition/1
  Pressure/1 -> Rate Transition1/1
  Rate Transition/1 -> Add/2
  Add/1 -> temperature/1
  Rate Transition1/1 -> pressure/1
  Band-Limited White Noise1/1 -> Add/1

== matlab function multi_model2015a/Control System/MATLAB Function ==
  data: p input; q input; r input; ax input; ay input; az input; Roll_Angle output; Pitch_Angle output; Yaw_Angle output
function [Roll_Angle, Pitch_Angle, Yaw_Angle] = sensor_fusion(p, q, r, ax, ay, az)

%================================Constants=================================

delta_t = 0.01;
degrees = 180 / pi;
radians = pi / 180;

%Attitude Estimator
Q_gyroBias = 0.000000087;           % Q_gyroBias: gyroscope noise
Q_angle = 0.000039;                 % Q_angle: accelerometer noise
R_angle = 20;                       % R_angle: high ==> gyroscope, low ==> accelerometer

%=============================Intitialization==============================

persistent initialize angle_roll bias1 P1 K1 phi angle_pitch bias2 P2 K2 theta angle_yaw;
    
if isempty(initialize)
    if isempty(angle_roll)
        angle_roll = 0;
        bias1 = 0;
        P1 = zeros(2);
        K1 = zeros([2,1]);
        phi = 0;
    end
    if isempty(angle_pitch)
        angle_pitch = 0;
        bias2 = 0;
        P2 = zeros(2);
        K2 = zeros([2,1]);
        theta = 0;
    end
    if isempty(angle_yaw)
        angle_yaw = 0;
    end
    initialize = 1;
else
    
%==============================Kalman Filter===============================

%--------------------------------Roll Angle--------------------------------

    Rate_Roll = p + (q * sin(phi) + r * cos(phi)) * tan(theta) - bias1;                     
    angle_roll = angle_roll + Rate_Roll * delta_t;                                          %Projected State (integrated gyro data)
    earth_roll = -atan(ay / az) * degrees;                                                  %Measurement Update (gravity vector)
    P1(1,1) = P1(1,1) + delta_t * (P1(2,2) * delta_t - P1(1,2) - P1(2,1) + Q_angle);        %Projected error covariance
    P1(1,2) = P1(1,2) - P1(2,2) * delta_t;
    P1(2,1) = P1(2,1) - P1(2,2) * delta_t;
    P1(2,2) = P1(2,2) + Q_gyroBias * delta_t;
    S1 = P1(1,1) + R_angle;                                                                 %Kalman Gain
    K1(1) = P1(1,1) / S1;
    K1(2) = P1(2,1) / S1;
    Y1 = earth_roll - angle_roll;                                                           %Estimate Update
    angle_roll = angle_roll + K1(1) * Y1;
    bias1 = bias1 + K1(2) * Y1;
    P1(1,1) = P1(1,1) - K1(1) * P1(1,1);                                                    %Update Error Covariance
    P1(1,2) = P1(1,2) - K1(1) * P1(1,2);
    P1(2,1) = P1(2,1) - K1(2) * P1(1,1);
    P1(2,2) = P1(2,2) - K1(2) * P1(1,2);
    phi = angle_roll * radians;
 
%--------------------------------Pitch Angle-------------------------------

    Rate_Pitch = q * cos(phi) + r * sin(phi) - bias2;                           
    angle_pitch = angle_pitch + Rate_Pitch * delta_t;                                       %Projected State (integrated gyro data)
    earth_pitch = atan(ax / az) * degrees;                                                  %Measurement Update (gravity vector)
    P2(1,1) = P2(1,1) + delta_t * (P2(2,2) * delta_t - P2(1,2) - P2(2,1) + Q_angle);        %Projected error covariance
    P2(1,2) = P2(1,2) - P2(2,2) * delta_t;
    P2(2,1) = P2(2,1) - P2(2,2) * delta_t;
    P2(2,2) = P2(2,2) + Q_gyroBias * delta_t;
    S2 = P2(1,1) + R_angle;                                                                 %Kalman Gain
    K2(1) = P2(1,1) / S2;
    K2(2) = P2(2,1) / S2;
    Y2 = earth_pitch - angle_pitch;                                                         %Estimate Update
    angle_pitch = angle_pitch + K2(1) * Y2;
    bias2 = bias2 + K2(2) * Y2;
    P2(1,1) = P2(1,1) - K2(1) * P2(1,1);                                                    %Update Error Covariance
    P2(1,2) = P2(1,2) - K2(1) * P2(1,2);
    P2(2,1) = P2(2,1) - K2(2) * P2(1,1);
    P2(2,2) = P2(2,2) - K2(2) * P2(1,2);
    theta = angle_pitch * radians;
    
%--------------------------------Yaw Angle---------------------------------

    angle_yaw = angle_yaw + (q * sin(phi) + r * cos(phi)) * sec(theta) * delta_t;           %Integrated gyro data

end

Roll_Angle = phi;
Pitch_Angle = theta;
Yaw_Angle = angle_yaw * radians/(2*pi);
    
%==========================================================================

== matlab function multi_model2015a/Control System/Waypoint Controller/MATLAB Function ==
  data: currentPosition input; WP input; status input; currentWP output
function currentWP = currentWP(currentPosition, WP, status)
%=============================Intitialization==============================
persistent initialize index sizeWPArray;
    
if isempty(initialize)
    if isempty(index)
        index = 1;       
    end    
    sizeWPArray = length(WP(:,1));  
    initialize = 1;
else
    if(status == 0)
        if((norm(-transpose(currentPosition) + WP(index,:)) < 0.1) && (index < sizeWPArray))
        index = index + 1;
        end   
    end
end
currentWP = WP(index,:);

== matlab function multi_model2015a/Control System/Position Controller/pwm_out1 ==
  data: accel_right input; curr_pitch input; roll_target output
function roll_target  = accel2roll_target(accel_right, curr_pitch)
roll_target = atan(accel_right*cos(curr_pitch) / 9.81);

== matlab function multi_model2015a/Dynamic Model/aircraft_dynamics ==
  data: pwm input; forces output; moments output; DCM input; p input; Vb input
function [forces, moments] = dynamics(pwm, DCM, p, Vb)

%================================Constants=================================

radsec = 0.104719755;
gravity = 9.81;
radians = pi / 180;

% Aircraft Parameters
motor_thrust = 1.450;                 % Maximum thrust of a single motor      (kg)
motor_constant = 470;               % Motor revolutions per volt            (KV)
motor_voltage = 22.2;               % Nominal motor voltage                 (V)
motor_efficiency = 0.8;             % Effective velocity
rotor_diameter = 0.254;              % Diameter of the rotor                 (meters)
aircraft_mass = 2.5;                % Aircraft mass                         (kg)
aircraft_diameter = 0.80;           % Motor to motor distance               (meters)
aircraft_dihedral = 0;              % Angle from base to arm                (degrees)
aircraft_mixer = 3;                 % Rotor position and rotation
% Quad [X] = 0
% Quad [+] = 1
% Hex  [X] = 2

%==============================Inertia Tensor==============================
% Octocopter BKAerohelper [+] 
%==============================Initialization==============================

persistent initialize;

g = [0; 0; gravity];
t = zeros(1, 8);

if isempty(initialize)
    DCM = zeros(3);
    initialize = 1;
end

for n = 1:8
    t(n) = (pwm(n) - 1000) / 1000;
end

%=================================Actuators================================

% [enabled, x(roll), y(pitch), z(yaw)]

M = zeros(8, 4);

if aircraft_mixer == 0
    M(1, :) = [1;  1;  1; -1];
    M(2, :) = [1, -1,  1,  1];
    M(3, :) = [1, -1, -1, -1];
    M(4, :) = [1,  1, -1,  1];
    M(5, :) = [0,  0,  0,  0];
    M(6, :) = [0,  0,  0,  0];
    M(7, :) = [0,  0,  0,  0];
    M(8, :) = [0,  0,  0,  0];
elseif aircraft_mixer == 1
    M(1, :) = [1;  0;  1; -1];
    M(2, :) = [1, -1,  0,  1];
    M(3, :) = [1,  0, -1, -1];
    M(4, :) = [1,  1,  0,  1];
    M(5, :) = [0,  0,  0,  0];
    M(6, :) = [0,  0,  0,  0];
    M(7, :) = [0,  0,  0,  0];
    M(8, :) = [0,  0,  0,  0];
elseif aircraft_mixer == 2
    M(1, :) = [1;  1;  1; -1];
    M(2, :) = [1, -1,  1,  1];
    M(3, :) = [1, -1,  0, -1];
    M(4, :) = [1, -1, -1,  1];
    M(5, :) = [1,  1, -1, -1];
    M(6, :) = [1,  1,  0,  1];
    M(7, :) = [0,  0,  0,  0];
    M(8, :) = [0,  0,  0,  0];
elseif aircraft_mixer == 3   %Octa +
    M(1, :) = [1;  0; -1; -1];
    M(2, :) = [1,  0,  1, -1];
    M(3, :) = [1, -sqrt(2)/2, -sqrt(2)/2, 1];
    M(4, :) = [1, -sqrt(2)/2,  sqrt(2)/2, 1];
    M(5, :) = [1,  sqrt(2)/2, -sqrt(2)/2, 1];
    M(6, :) = [1,  sqrt(2)/2,  sqrt(2)/2, 1];
    M(7, :) = [1,  1,  0, -1];
    M(8, :) = [1, -1,  0, -1];
else
    M(1, :) = [0;  0;  0;  0];
    M(2, :) = [0,  0,  0,  0];
    M(3, :) = [0,  0,  0,  0];
    M(4, :) = [0,  0,  0,  0];
    M(5, :) = [0,  0,  0,  0];
    M(6, :) = [0,  0,  0,  0];
    M(7, :) = [0,  0,  0,  0];
    M(8, :) = [0,  0,  0,  0];
end

%==================================Forces==================================

F_z = zeros(1, 8);

for n = 1:8
    F_z(n) = t(n) * motor_thrust * gravity * M(n, 1)...                     % rotor forces
        * sin((90 - aircraft_dihedral) * radians);
end

A = [rotor_diameter * 0.01,...                                              % rotor cross sectional area
    aircraft_diameter ^ 2 / 10,...                                          % body cross sectional area (X)
    aircraft_diameter ^ 2 / 10,...                                          % body cross sectional area (Y)
    pi * ((aircraft_diameter - rotor_diameter) / 2) ^ 2];                   % body cross sectional area (Z)

F_d = zeros(1, 3);

for n = 1:3
    F_d(n) = p / 2 * A(n + 1) * (Vb(n)) ^ 2;
    if Vb(n) > 0
        F_d(n) = F_d(n) * -1;
    end
end

forces = zeros(3, 1);

F_g = aircraft_mass .* (DCM * g);                                           % gravitational force
forces(1) =  F_g(1) + F_d(1);
forces(2) =  F_g(2) + F_d(2);
forces(3) =  F_g(3) - sum(F_z) + 2 * F_d(3);

%==================================Moments=================================

m = zeros(8, 4);

for n = 1:8
    m(n, :) = F_z(n) .* M(n, :);
end

m = (aircraft_diameter / 2) .* m;                                           % x & y moments

K = motor_constant * motor_voltage * motor_efficiency * radsec;
Vr = zeros(1, 8);

for n = 1:8
    Vr(n) = t(n) * K;                                                       % rotor angular velocity
end

d = zeros(1, 8);

for n = 1:8
    d(n) =  M(n, 4) * p / 2 * A(1) * (Vr(n) * rotor_diameter / 10) ^ 2;     % aerodynamic drag force of the rotor
end

T = zeros(1, 8);

for n = 1:8
    T(n) = d(n);                                                            % total rotor torque
end

moments = zeros(3, 1);

moments(1) = sum(m(:, 2));
moments(2) = sum(m(:, 3));
moments(3) = sum(T);

%==========================================================================

== matlab function multi_model2015a/Control System/Position Controller/pwm_out2 ==
  data: pitch_target output; accel_forward input
function pitch_target  = accel2pitch_target(accel_forward)
pitch_target = atan(-accel_forward / 9.81);

== matlab function multi_model2015a/Control System/pwm_out ==
  data: Roll input; M1 output; Pitch input; Thrust input; Yaw input; M2 output; M3 output; M4 output; M5 output; M6 output; M7 output; M8 output
function [M1, M2, M3, M4, M5, M6, M7, M8] = motor_mixer(Roll, Pitch, Thrust, Yaw)

%===========================Settings & Constants===========================

idle_PWM = 1122;
aircraft_mixer = 3;
% Quad [X] = 0
% Quad [+] = 1
% Hex  [X] = 2

%===============================Quad X Mixer===============================

if aircraft_mixer == 0;        % Quad X
    M1 = ((Roll + Pitch - Yaw) * Thrust / 2 + Thrust) * 800 + idle_PWM;
    M2 = ((-Roll + Pitch + Yaw) * Thrust / 2 + Thrust) * 800 + idle_PWM;
    M3 = ((-Roll - Pitch - Yaw) * Thrust / 2 + Thrust) * 800 + idle_PWM;
    M4 = ((Roll - Pitch + Yaw) * Thrust / 2 + Thrust) * 800 + idle_PWM;
    M5 = 1122;
    M6 = 1122;
    M7 = 1122;
    M8 = 1122;
elseif aircraft_mixer == 1;    % Quad +
    M1 = ((Pitch - Yaw) * Thrust / 2 + Thrust) * 800 + idle_PWM;
    M2 = ((-Roll + Yaw) * Thrust / 2 + Thrust) * 800 + idle_PWM;
    M3 = ((-Pitch - Yaw) * Thrust / 2 + Thrust) * 800 + idle_PWM;
    M4 = ((Roll + Yaw) * Thrust / 2 + Thrust) * 800 + idle_PWM;
    M5 = 1122;
    M6 = 1122;
    M7 = 1122;
    M8 = 1122;
elseif aircraft_mixer == 2;    % Hex X
    M1 = ((Pitch + Roll / 2 - Yaw) * Thrust / 2 + Thrust) * 800 + idle_PWM;
    M2 = ((Pitch - Roll / 2 + Yaw) * Thrust / 2 + Thrust) * 800 + idle_PWM;
    M3 = ((-Roll - Yaw) * Thrust / 2 + Thrust) * 800 + idle_PWM;
    M4 = ((-Pitch - Roll / 2 + Yaw) * Thrust / 2 + Thrust) * 800 + idle_PWM;
    M5 = ((-Pitch + Roll / 2 - Yaw) * Thrust / 2 + Thrust) * 800 + idle_PWM;
    M6 = ((Roll + Yaw) * Thrust / 2 + Thrust) * 800 + idle_PWM;
    M7 = 1122;
    M8 = 1122;
elseif aircraft_mixer == 3;    % Octa +
    M1 = ((-Pitch - Yaw)* Thrust / 8 + Thrust)* 800 + idle_PWM;    
    M2 = (( Pitch - Yaw)* Thrust / 8 + Thrust)* 800 + idle_PWM;
    M3 = (((-Pitch - Roll)* sqrt(2)/2 + Yaw)* Thrust / 8 + Thrust)* 800 + idle_PWM;    
    M4 = ((( Pitch - Roll)* sqrt(2)/2 + Yaw)* Thrust / 8 + Thrust)* 800 + idle_PWM;    
    M5 = (((-Pitch + Roll)* sqrt(2)/2 + Yaw)* Thrust / 8 + Thrust)* 800 + idle_PWM;    
    M6 = ((( Pitch + Roll)* sqrt(2)/2 + Yaw)* Thrust / 8 + Thrust)* 800 + idle_PWM;    
    M7 = (( Roll - Yaw)* Thrust / 8 + Thrust)* 800 + idle_PWM;
    M8 = ((-Roll - Yaw)* Thrust / 8 + Thrust)* 800 + idle_PWM;
else
    M1 = 1122;
    M2 = 1122;
    M3 = 1122;
    M4 = 1122;
    M5 = 1122;
    M6 = 1122;
    M7 = 1122;
    M8 = 1122;
end
%==========================================================================

== matlab function multi_model2015a/Signal Receiver/MATLAB Function ==
  data: WPdataTable output
function WPdataTable = getWP()
WPdataTable = [0 0 5; 0 3 5; 4 3 5; 0 0 5; 0 0 2];
% WPdataTable = [0 0 5; 0 0 3; 0 0 5];
